simulink model "Integration_1_1"  (R2024b)
settings: Solver=VariableStepAuto  StartTime=0.0  StopTime=4  RelTol=1e-3
undefined symbols (not defined in the file): Ion, Lithium, Ts_Control
libraries: ee_lib x30, nesl_utility x24, spsSeriesRLCBranchLib x22, simulink x21, slpidlib x18, spsParallelRLCBranchLib x18, spsCurrentVoltageSimscapeInterfaceLib x18, powerlib_extras x18, spsThreePhaseVIMeasurementLib x7, spsGroundLib x7, spsThreePhaseSeriesRLCBranchLib x7, spsBoostConverterLib x6
(part 5 of 5)

== system Integration_1_1/VSC Control5/Uabc_ref Generation max (m) = 1 ==
  note: (Correction for transformer
      |  D1 connection)
  note: (Correction for delai of Ts_Control)
  wt : Inport
  VdVq_conv : Inport  Port=2
  Add1 : Sum  Inputs=++++
  Add2 : Sum
  Complex to Magnitude-Angle : ComplexToMagnitudeAngle
  Constant : Constant  Value=-pi/6
  Constant1 : Constant  Value=Vnom_dc
  Constant2 : Constant  Value="[ 0  -2*pi/3  2*pi/3  ]"
  Constant3 : Constant  Value=Vnom_sec*sqrt(2)/sqrt(3)
  Constant4 : Constant  Value=Ts*Fnom*(2*pi)
  Demux1 : Demux  Outputs=2
  Gain1 : Gain  Gain=1/2
  Product : Product  Inputs=*/  RndMeth=Zero
  Product1 : Product  Inputs=*/  RndMeth=Zero
  Product2 : Product  Inputs=**  RndMeth=Zero
  Real-Imag to Complex : RealImagToComplex
  Saturation : Saturate  UpperLimit=1  LowerLimit=0
  Trigonometric Function : Trigonometry
  Uabc_ref : Outport  VectorParamsAs1DForOutWhenUnconnected=off
  wires:
  Complex to Magnitude-Angle/1 -> Saturation/1
  Constant1/1 -> Gain1/1
  VdVq_conv/1 -> Product1/1
  Product1/1 -> Demux1/1
  Gain1/1 -> Product/1
  Real-Imag to Complex/1 -> Complex to Magnitude-Angle/1
  Demux1/1 -> Real-Imag to Complex/1
  Demux1/2 -> Real-Imag to Complex/2
  Constant2/1 -> Add1/2
  Constant/1 -> Add1/3
  Constant3/1 -> Product/2
  Product/1 -> Product1/2
  Complex to Magnitude-Angle/2 -> Add2/1
  Add1/1 -> Add2/2
  Add2/1 -> Trigonometric Function/1
  Saturation/1 -> Product2/1
  Trigonometric Function/1 -> Product2/2
  Product2/1 -> Uabc_ref/1
  wt/1 -> Add1/1
  Constant4/1 -> Add1/4

== system Integration_1_1/VSC Control5/VDC Regulator ==
  Vdc_meas : Inport  PortDimensions=1
  Vdc_ref : Inport  Port=2  PortDimensions=1
  PI : slpidlib/PID Controller  Controller=PI  Form=Parallel  TimeDomain=Discrete-time  UseExternalTs=off  SampleTime=Ts  IntegratorMethod=Trapezoidal  FilterMethod=Forward Euler  ControllerParametersSource=internal  P=Kp_VDCreg  I=Ki_VDCreg  UseKiTs=off  D=0  UseExternalDerivativeSource=off  N=100  UseFilter=on  TunerSelectOption=Transfer Function Based (PID Tuner App)  InitialConditionSource=internal  InitialConditionForIntegrator=0  InitialConditionForFilter=0  DifferentiatorICPrevScaledInput=0  ExternalReset=none  TrackingMode=off  Kt=1  LimitOutput=on  SatLimitsSource=internal  UpperSaturationLimit=1.5  LowerSaturationLimit=-1.5  LinearizeAsGain=off  AntiWindupMode=none  Kb=1  LimitIntegrator=off  UpperIntegratorSaturationLimit=inf  LowerIntegratorSaturationLimit=-inf  POutMin=[]  POutMax=[]  IOutMin=[]  IOutMax=[]  DOutMin=[]  DOutMax=[]  NOutMin=[]  NOutMax=[]  SumOutMin=[]  SumOutMax=[]  SaturationOutMin=[]  SaturationOutMax=[]  PParamMin=[]  PParamMax=[]  IParamMin=[]  IParamMax=[]  DParamMin=[]  DParamMax=[]  NParamMin=[]  NParamMax=[]  KbParamMin=[]  KbParamMax=[]  KtParamMin=[]  KtParamMax=[]  KbOutMin=[]  KbOutMax=[]  KtOutMin=[]  KtOutMax=[]  IntegratorOutMin=[]  IntegratorOutMax=[]  FilterOutMin=[]  FilterOutMax=[]  SumI1OutMin=[]  SumI1OutMax=[]  SumI2OutMin=[]  SumI2OutMax=[]  SumI3OutMin=[]  SumI3OutMax=[]  SumI4OutMin=[]  SumI4OutMax=[]  SumDOutMin=[]  SumDOutMax=[]  DifferentiatorOutMin=[]  DifferentiatorOutMax=[]  FilterDiffOutCoefMin=[]  FilterDiffOutCoefMax=[]  ReciprocalOutMin=[]  ReciprocalOutMax=[]  SumDenOutMin=[]  SumDenOutMax=[]  SumNumOutMin=[]  SumNumOutMax=[]  DivideOutMin=[]  DivideOutMax=[]  UdiffTsProdOutMin=[]  UdiffTsProdOutMax=[]  NTsProdOutMin=[]  NTsProdOutMax=[]  UintegralTsProdOutMin=[]  UintegralTsProdOutMax=[]  UngainTsProdOutMin=[]  UngainTsProdOutMax=[]  ClampingZeroOutDataTypeStr=Inherit: Inherit via back propagation  ClampingZeroOutMin=[]  ClampingZeroOutMax=[]  FilterDenConstantOutDataTypeStr=Inherit: Inherit via back propagation  FilterDenConstantOutMin=[]  FilterDenConstantOutMax=[]  PCopyOutDataTypeStr=Inherit: Inherit via back propagation  PCopyOutMin=[]  PCopyOutMax=[]  NCopyOutDataTypeStr=Inherit: Inherit via back propagation  NCopyOutMin=[]  NCopyOutMax=[]  IntegratorContinuousStateAttributes=''  IntegratorStateMustResolveToSignalObject=off  IntegratorRTWStateStorageClass=Auto  FilterContinuousStateAttributes=''  FilterStateMustResolveToSignalObject=off  FilterRTWStateStorageClass=Auto  ParallelPVariant=InternalParameters  IdealPVariant=Disabled  IVariant=InternalParameters  DVariant=Disabled  IntegratorVariant=Discrete  SatVariant=Enabled  AWVariant=Passthrough  PCopyVariant=Disabled  TRVariant=Disabled  FdbkBlocksVariant=Forward  IdealPFdbkVariant=Disabled  SatFdbkVariant=Disabled  DerivativeFilterVariant=Disabled  NVariant=Disabled  NCopyVariant=Disabled_SignalSpec  FilterICVariant=Disabled  IntegratorICVariant=InternalICs  ExternalResetVariant=Disabled  TRSumVariant=Passthrough  SumFdbkVariant=Disabled  SumVariant=Sum_PI  TsampFilterVariant=InternalTs  TsampNgainVariant=Passthrough  TsampIntegralVariant=Disabled_SignalSpec  ExternalSaturationOutDataTypeStr=Inherit: Same as second input  DerivativeSourceVariant=Disabled  PreIntVariant=InternalPreInt
  Rtot_pu3 : Gain  Gain=1/Vnom_dc  SaturateOnIntegerOverflow=on  OutDataTypeStr=Inherit: Same as input  ParamDataTypeStr=Inherit: Same as input
  Sum : Sum  Inputs=|+-
  Id_ref : Outport  SampleTime=Ts  InitialOutput=0  VectorParamsAs1DForOutWhenUnconnected=off
  wires:
  PI/1 -> Id_ref/1
  Sum/1 -> Rtot_pu3/1
  Vdc_meas/1 -> Sum/1
  Vdc_ref/1 -> Sum/2
  Rtot_pu3/1 -> PI/1

== matlab function Integration_1_1/Subsystem9/MPPT3/MATLAB Function1 ==
  data: ipv input; Vref output; vpv input
function Vref = incCondMPPT(ipv, vpv)
%#codegen
% Incremental Conductance MPPT – returns updated reference voltage Vref

% Persistent variables
persistent Iprev Vprev Vref_prev

% Initialize persistent variables
if isempty(Iprev)
    Iprev = ipv;
    Vprev = vpv;
    Vref_prev = vpv;  % Initialize at first voltage sample
end

% Output initialization (helps Simulink infer output type/size)
Vref = 0;

% Parameters
STEP = 1;      % Voltage adjustment step (V)
TOL  = 1e-4;     % Tolerance for MPP detection
V_MIN = 5;       % Minimum PV voltage

% Handle invalid conditions
if isnan(ipv) || isnan(vpv) || vpv < V_MIN
    Vref = Vref_prev;
    return;
end

% Compute deltas
dI = ipv - Iprev;
dV = vpv - Vprev;

% MPPT logic
if abs(dV) < 1e-6
    if dI > TOL
        Vref = Vref_prev + STEP;
    elseif dI < -TOL
        Vref = Vref_prev - STEP;
    else
        Vref = Vref_prev;
    end
else
    incCond = dI / dV;
    instCond = -ipv / vpv;

    if abs(incCond - instCond) < TOL
        Vref = Vref_prev;
    elseif incCond > instCond
        Vref = Vref_prev + STEP;
    else
        Vref = Vref_prev - STEP;
    end
end

% Clamp to minimum safe voltage
Vref = max(Vref, V_MIN);

% Update persistent variables
Iprev = ipv;
Vprev = vpv;
Vref_prev = Vref;
end

== matlab function Integration_1_1/Subsystem13/MPPT4/MATLAB Function1 ==
  data: ipv input; Vref output; vpv input
function Vref = incCondMPPT(ipv, vpv)
%#codegen
% Incremental Conductance MPPT – returns updated reference voltage Vref

% Persistent variables
persistent Iprev Vprev Vref_prev

% Initialize persistent variables
if isempty(Iprev)
    Iprev = ipv;
    Vprev = vpv;
    Vref_prev = vpv;  % Initialize at first voltage sample
end

% Output initialization (helps Simulink infer output type/size)
Vref = 0;

% Parameters
STEP = 1.5;      % Voltage adjustment step (V)
TOL  = 1e-4;     % Tolerance for MPP detection
V_MIN = 5;       % Minimum PV voltage

% Handle invalid conditions
if isnan(ipv) || isnan(vpv) || vpv < V_MIN
    Vref = Vref_prev;
    return;
end

% Compute deltas
dI = ipv - Iprev;
dV = vpv - Vprev;

% MPPT logic
if abs(dV) < 1e-6
    if dI > TOL
        Vref = Vref_prev + STEP;
    elseif dI < -TOL
        Vref = Vref_prev - STEP;
    else
        Vref = Vref_prev;
    end
else
    incCond = dI / dV;
    instCond = -ipv / vpv;

    if abs(incCond - instCond) < TOL
        Vref = Vref_prev;
    elseif incCond > instCond
        Vref = Vref_prev + STEP;
    else
        Vref = Vref_prev - STEP;
    end
end

% Clamp to minimum safe voltage
Vref = max(Vref, V_MIN);

% Update persistent variables
Iprev = ipv;
Vprev = vpv;
Vref_prev = Vref;
end

== matlab function Integration_1_1/Subsystem/MPPT/MATLAB Function1 ==
  data: ipv input; Vref output; vpv input
function Vref = incCondMPPT(ipv, vpv)
%#codegen
% Incremental Conductance MPPT – returns updated reference voltage Vref

% Persistent variables
persistent Iprev Vprev Vref_prev

% Initialize persistent variables
if isempty(Iprev)
    Iprev = ipv;
    Vprev = vpv;
    Vref_prev = vpv;  % Initialize at first voltage sample
end

% Output initialization (helps Simulink infer output type/size)
Vref = 0;

% Parameters
STEP = 1.5;      % Voltage adjustment step (V)
TOL  = 1e-4;     % Tolerance for MPP detection
V_MIN = 5;       % Minimum PV voltage

% Handle invalid conditions
if isnan(ipv) || isnan(vpv) || vpv < V_MIN
    Vref = Vref_prev;
    return;
end

% Compute deltas
dI = ipv - Iprev;
dV = vpv - Vprev;

% MPPT logic
if abs(dV) < 1e-6
    if dI > TOL
        Vref = Vref_prev + STEP;
    elseif dI < -TOL
        Vref = Vref_prev - STEP;
    else
        Vref = Vref_prev;
    end
else
    incCond = dI / dV;
    instCond = -ipv / vpv;

    if abs(incCond - instCond) < TOL
        Vref = Vref_prev;
    elseif incCond > instCond
        Vref = Vref_prev + STEP;
    else
        Vref = Vref_prev - STEP;
    end
end

% Clamp to minimum safe voltage
Vref = max(Vref, V_MIN);

% Update persistent variables
Iprev = ipv;
Vprev = vpv;
Vref_prev = Vref;
end

== matlab function Integration_1_1/Subsystem2/MPPT2/MATLAB Function1 ==
  data: ipv input; Vref output; vpv input
function Vref = incCondMPPT(ipv, vpv)
%#codegen
% Incremental Conductance MPPT – returns updated reference voltage Vref

% Persistent variables
persistent Iprev Vprev Vref_prev

% Initialize persistent variables
if isempty(Iprev)
    Iprev = ipv;
    Vprev = vpv;
    Vref_prev = vpv;  % Initialize at first voltage sample
end

% Output initialization (helps Simulink infer output type/size)
Vref = 0;

% Parameters
STEP = 1.5;      % Voltage adjustment step (V)
TOL  = 1e-4;     % Tolerance for MPP detection
V_MIN = 5;       % Minimum PV voltage

% Handle invalid conditions
if isnan(ipv) || isnan(vpv) || vpv < V_MIN
    Vref = Vref_prev;
    return;
end

% Compute deltas
dI = ipv - Iprev;
dV = vpv - Vprev;

% MPPT logic
if abs(dV) < 1e-6
    if dI > TOL
        Vref = Vref_prev + STEP;
    elseif dI < -TOL
        Vref = Vref_prev - STEP;
    else
        Vref = Vref_prev;
    end
else
    incCond = dI / dV;
    instCond = -ipv / vpv;

    if abs(incCond - instCond) < TOL
        Vref = Vref_prev;
    elseif incCond > instCond
        Vref = Vref_prev + STEP;
    else
        Vref = Vref_prev - STEP;
    end
end

% Clamp to minimum safe voltage
Vref = max(Vref, V_MIN);

% Update persistent variables
Iprev = ipv;
Vprev = vpv;
Vref_prev = Vref;
end

== matlab function Integration_1_1/Subsystem15/MPPT5/MATLAB Function1 ==
  data: ipv input; Vref output; vpv input
function Vref = incCondMPPT(ipv, vpv)
%#codegen
% Incremental Conductance MPPT – returns updated reference voltage Vref

% Persistent variables
persistent Iprev Vprev Vref_prev

% Initialize persistent variables
if isempty(Iprev)
    Iprev = ipv;
    Vprev = vpv;
    Vref_prev = vpv;  % Initialize at first voltage sample
end

% Output initialization (helps Simulink infer output type/size)
Vref = 0;

% Parameters
STEP = 1.5;      % Voltage adjustment step (V)
TOL  = 1e-4;     % Tolerance for MPP detection
V_MIN = 5;       % Minimum PV voltage

% Handle invalid conditions
if isnan(ipv) || isnan(vpv) || vpv < V_MIN
    Vref = Vref_prev;
    return;
end

% Compute deltas
dI = ipv - Iprev;
dV = vpv - Vprev;

% MPPT logic
if abs(dV) < 1e-6
    if dI > TOL
        Vref = Vref_prev + STEP;
    elseif dI < -TOL
        Vref = Vref_prev - STEP;
    else
        Vref = Vref_prev;
    end
else
    incCond = dI / dV;
    instCond = -ipv / vpv;

    if abs(incCond - instCond) < TOL
        Vref = Vref_prev;
    elseif incCond > instCond
        Vref = Vref_prev + STEP;
    else
        Vref = Vref_prev - STEP;
    end
end

% Clamp to minimum safe voltage
Vref = max(Vref, V_MIN);

% Update persistent variables
Iprev = ipv;
Vprev = vpv;
Vref_prev = Vref;
end

== matlab function Integration_1_1/Subsystem18/MPPT6/MATLAB Function1 ==
  data: ipv input; Vref output; vpv input
function Vref = incCondMPPT(ipv, vpv)
%#codegen
% Incremental Conductance MPPT – returns updated reference voltage Vref

% Persistent variables
persistent Iprev Vprev Vref_prev

% Initialize persistent variables
if isempty(Iprev)
    Iprev = ipv;
    Vprev = vpv;
    Vref_prev = vpv;  % Initialize at first voltage sample
end

% Output initialization (helps Simulink infer output type/size)
Vref = 0;

% Parameters
STEP = 1.5;      % Voltage adjustment step (V)
TOL  = 1e-4;     % Tolerance for MPP detection
V_MIN = 5;       % Minimum PV voltage

% Handle invalid conditions
if isnan(ipv) || isnan(vpv) || vpv < V_MIN
    Vref = Vref_prev;
    return;
end

% Compute deltas
dI = ipv - Iprev;
dV = vpv - Vprev;

% MPPT logic
if abs(dV) < 1e-6
    if dI > TOL
        Vref = Vref_prev + STEP;
    elseif dI < -TOL
        Vref = Vref_prev - STEP;
    else
        Vref = Vref_prev;
    end
else
    incCond = dI / dV;
    instCond = -ipv / vpv;

    if abs(incCond - instCond) < TOL
        Vref = Vref_prev;
    elseif incCond > instCond
        Vref = Vref_prev + STEP;
    else
        Vref = Vref_prev - STEP;
    end
end

% Clamp to minimum safe voltage
Vref = max(Vref, V_MIN);

% Update persistent variables
Iprev = ipv;
Vprev = vpv;
Vref_prev = Vref;
end

== matlab function Integration_1_1/Subsystem1/BATT chg-dshg logic1/MATLAB Function1 ==
  data: Vdc input; Vbatt input; I_batt_meas input; I_batt_ref_mag input; D output; mode input
% MATLAB implementation of unified PI control for bidirectional DC-DC converter
% Modified to allow manual toggle between charging (mode = 0) and discharging (mode = 1)

function D = bidirectional_controller(Vdc, Vbatt, I_batt_meas, I_batt_ref_mag, mode)
%#codegen

% Limits
Imax_charge = 50;
Imax_discharge = -50;

% PI gains
Kp = 0.9;
Ki = 0.5;
persistent integral_error
if isempty(integral_error)
    integral_error = 0;
end

% Adjust reference sign based on mode
if mode == 0
    I_batt_ref = I_batt_ref_mag;      % Charging
elseif mode == 1
    I_batt_ref = -I_batt_ref_mag;     % Discharging
else
    I_batt_ref = 0;
end

% Clamp current reference
I_batt_ref = max(min(I_batt_ref, Imax_charge), Imax_discharge);

% PI control
error = I_batt_ref - I_batt_meas;
dt = 1e-4;
integral_error = integral_error + error * dt;
PI_output = Kp * error + Ki * integral_error;

% Base duty calculation
if mode == 0
    D_base = Vbatt / Vdc;             % Buck mode
elseif mode == 1
    D_base = 1 - Vbatt / Vdc;         % Boost mode
else
    D_base = 0;
end

% Total duty
D = D_base + PI_output;
D = min(max(D, 0.05), 0.95);

end
